simulink model "scattering_FP"  (R2021b)
settings: Solver=ode45  StartTime=0.0  StopTime=10  FixedStep=Ts  MinStep=1e-5  RelTol=1e-5
undefined symbols (not defined in the file): A, Ak, B, b, Be, Bh, Bs, C, d, Dh, Discrete, Dm, Ds, Fc, Fip, Flp, Jh, Ke, Kh, Ks, Mm, Ms, noise, Ph, R, Time, Ts, x0, xe
libraries: simulink x3, ctrlSharedLib x2, cstblocks x1
settings Model: Creator=simon  LastModifiedBy=buse
settings SolverCC: AlgebraicLoopSolver=LineSearch
settings DebuggingCC: SFMachineParentedDataDiag=warning

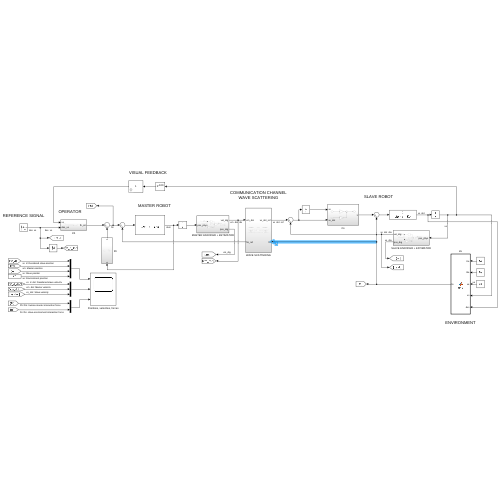
[thumbnail: Simulink's stored preview of the top-level diagram]
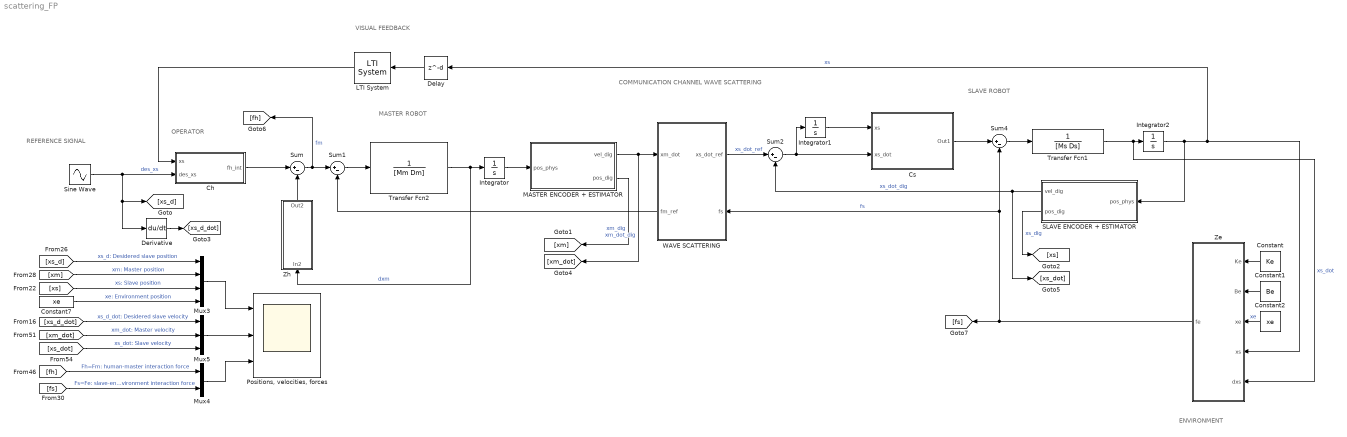
== system scattering_FP ==
  note: REFERENCE SIGNAL
  note: MASTER ROBOT
  note: COMMUNICATION CHANNEL
      | WAVE SCATTERING
  note: VISUAL FEEDBACK
  note: SLAVE ROBOT
  note: OPERATOR
  note: ENVIRONMENT
  Ch : Subsystem
  Constant : Constant  Value=Ke
  Constant1 : Constant  Value=Be
  Constant2 : Constant  Value=xe
  Constant7 : Constant  Value=xe
  Cs : Subsystem
  Delay : Delay  DelayLength=d
  Derivative : Derivative
  Integrator : Integrator
  Integrator1 : Integrator
  Integrator2 : Integrator
  LTI System : cstblocks/LTI System  sys=1  IC=[]
  MASTER ENCODER + ESTIMATOR : Subsystem
  Mux3 : Mux
  Mux4 : Mux  Inputs=2
  Mux5 : Mux  Inputs=3
  "Positions, velocities, forces" : Scope  NumInputPorts=3
  SLAVE ENCODER + ESTIMATOR : Subsystem
  Sine Wave : Sin  Amplitude=A  Frequency=Fc  SampleTime=0
  Sum{,1..2,4} (4 alike) : Sum  Inputs=|+-
  Transfer Fcn1 : TransferFcn  Denominator=[Ms Ds]
  Transfer Fcn2 : TransferFcn  Denominator=[Mm Dm]
  WAVE SCATTERING : Subsystem
      settings: PortSchema="{\"entries\":[{\"content\":{\"sides\":[{\"content\":{\"connectorIds\":[\"In1\",\"Out2\"]},\"type\":\"ConnectorPlacement.EquallySpacedRectSide\",\"uuid\":\"b52b5263-ec77-4a5b-a444-fedf8384a1f4\"},{\"content\":{\"connectorIds\":[\"Out1\",\"In2\"],\"side\":\"RIGHT\"},\"type\":\"ConnectorPlacement.EquallySpacedRectSide\",\"uuid\":\"29fc6d0d-53a2-4de5-b8fc-fdc6e2130f9a\"},{\"content\":{\"connectorIds\":[],\"side\":\"TOP\"},\"type\":\"ConnectorPlacement.EquallySpacedRectSide\",\"uuid\":\"d00abe1a-0b08-4fbd-831b-b235aed68611\"},{\"content\":{\"connectorIds\":[],\"side\":\"HIDDEN\"},\"type\":\"ConnectorPlacement.EquallySpacedRectSide\",\"uuid\":\"d0d3daa3-ebbf-4bb5-b3d9-7ef522d44ef5\"}]},\"type\":\"ConnectorPlacement.EquallySpacedConnector\",\"uuid\":\"e5a03f62-d534-4700-82c8-2ace6ee2abeb\"}],\"packageUris\":[\"http://schema.mathworks.com/mf0/Connector/R2020b\"],\"version\":\"1.0\"}"
  Ze : MATLAB Function  TreatAsAtomicUnit=on
  Zh : Subsystem
  wires:
  Zh/1(Out2) -> Sum/2
  Sum1/1 -> Transfer Fcn2/1
  Sum4/1 -> Transfer Fcn1/1
  Transfer Fcn1/1 -> Ze/5(dxs), Integrator2/1  "xs_dot"
  Integrator2/1 -> SLAVE ENCODER + ESTIMATOR/1(pos_phys), Ze/4(xs), Delay/1  "xs"
  Constant2/1 -> Ze/3(xe)  "xe"
  Constant1/1 -> Ze/2(Be)
  Constant/1 -> Ze/1(Ke)
  Sum/1 -> [fh], Sum1/1  "fm"
  WAVE SCATTERING/2(fm_ref) -> Sum1/2
  WAVE SCATTERING/1(xs_dot_ref) -> Sum2/1  "xs_dot_ref"
  Sum2/1 -> Integrator1/1, Cs/2(xs_dot)
  Integrator1/1 -> Cs/1(xs)
  Cs/1(Out1) -> Sum4/1
  MASTER ENCODER + ESTIMATOR/1(vel_dig) -> [xm_dot], WAVE SCATTERING/1(xm_dot)  "xm_dot_dig"
  Ch/1(fh_int) -> Sum/1
  LTI System/1 -> Ch/1(xs)
  SLAVE ENCODER + ESTIMATOR/1(vel_dig) -> [xs_dot], Sum2/2  "xs_dot_dig"
  Ze/1(fe) -> [fs], WAVE SCATTERING/2(fs), Sum4/2  "fs"
  Sine Wave/1 -> Derivative/1, [xs_d], Ch/2(des_xs)  "des_xs"
  Delay/1 -> LTI System/1
  [fs] -> Mux4/2  "Fs=Fe: slave-environment interaction force"
  [xm_dot] -> Mux5/2  "xm_dot: Master velocity"
  [xs_d] -> Mux3/1  "xs_d: Desidered slave position"
  [fh] -> Mux4/1  "Fh=Fm: human-master interaction force"
  [xs_dot] -> Mux5/3  "xs_dot: Slave velocity"
  [xs_d_dot] -> Mux5/1  "xs_d_dot: Desidered slave velocity"
  Mux5/1 -> "Positions, velocities, forces"/2
  Mux3/1 -> "Positions, velocities, forces"/1
  Mux4/1 -> "Positions, velocities, forces"/3
  [xm] -> Mux3/2  "xm: Master position"
  [xs] -> Mux3/3  "xs: Slave position"
  Constant7/1 -> Mux3/4  "xe: Environment position"
  MASTER ENCODER + ESTIMATOR/2(pos_dig) -> [xm]  "xm_dig"
  SLAVE ENCODER + ESTIMATOR/2(pos_dig) -> [xs]  "xs_dig"
  Derivative/1 -> [xs_d_dot]
  Transfer Fcn2/1 -> Integrator/1, Zh/1(In2)  "dxm"
  Integrator/1 -> MASTER ENCODER + ESTIMATOR/1(pos_phys)

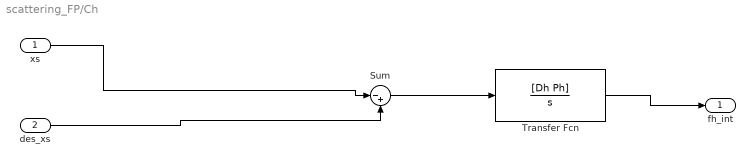
== system scattering_FP/Ch ==
  xs : Inport
  des_xs : Inport  Port=2
  Sum : Sum  Inputs=|-+
  Transfer Fcn : TransferFcn  Numerator=[Dh Ph]  Denominator=[1 0]
  fh_int : Outport
  wires:
  xs/1 -> Sum/1
  des_xs/1 -> Sum/2
  Sum/1 -> Transfer Fcn/1
  Transfer Fcn/1 -> fh_int/1

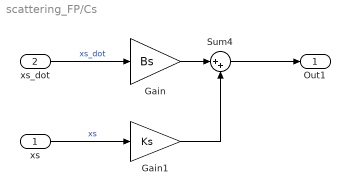
== system scattering_FP/Cs ==
  xs : Inport
  xs_dot : Inport  Port=2
  Gain : Gain  Gain=Bs
  Gain1 : Gain  Gain=Ks
  Sum4 : Sum  Inputs=|++
  Out1 : Outport
  wires:
  Gain1/1 -> Sum4/2
  Sum4/1 -> Out1/1
  xs_dot/1 -> Gain/1  "xs_dot"
  Gain/1 -> Sum4/1
  xs/1 -> Gain1/1  "xs"

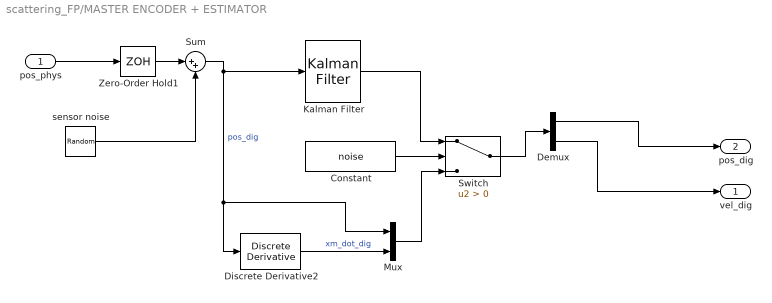
== system scattering_FP/MASTER ENCODER + ESTIMATOR ==
  pos_phys : Inport
  Constant : Constant  Value=noise
  Demux : Demux  Outputs=2
  Discrete Derivative2 : simulink/Discrete/Discrete Derivative  gainval=1.0  ICPrevScaledInput=0.0  OutMin=[]  OutMax=[]  OutDataType=fixdt(1, 16)  OutScaling=2^-10  DoSatur=off
  Kalman Filter : ctrlSharedLib/Kalman Filter  TimeDomain=Discrete-Time  UseCurrentEstimator=on  ModelSource=Individual A, B, C, D matrices  ModelSourceVariable=ss(0.95,1,1,0,1)  A=Ak  B=B  C=C  D=0  NumberOfStates=2  NumberOfInputs=1  NumberOfOutputs=1  InitialEstimateSource=Dialog  X0=x0  P0=10  UseK=off  UseGH=off  NumberOfProcessNoiseInputs=1  G=1  TimeInvariantG=on  H=0  TimeInvariantH=on  Q=Q_m  TimeInvariantQ=on  R=R  TimeInvariantR=on  N=0  TimeInvariantN=on  AddInputPort=off  AddEnablePort=off  OutputEstimatedY=off  OutputP=off  Ts=Ts
  Mux : Mux  Inputs=2
  Sum : Sum  Inputs=|++
  Switch : Switch  Criteria=u2 > Threshold
  Zero-Order Hold1 : ZeroOrderHold  SampleTime=Ts
  sensor noise : RandomNumber  Variance=noise  SampleTime=Ts
  vel_dig : Outport
  pos_dig : Outport  Port=2
  wires:
  pos_phys/1 -> Zero-Order Hold1/1
  Zero-Order Hold1/1 -> Sum/1
  sensor noise/1 -> Sum/2
  Kalman Filter/1 -> Switch/1
  Sum/1 -> Mux/1, Discrete Derivative2/1, Kalman Filter/1  "pos_dig"
  Constant/1 -> Switch/2
  Mux/1 -> Switch/3
  Discrete Derivative2/1 -> Mux/2  "xm_dot_dig"
  Switch/1 -> Demux/1
  Demux/1 -> pos_dig/1
  Demux/2 -> vel_dig/1

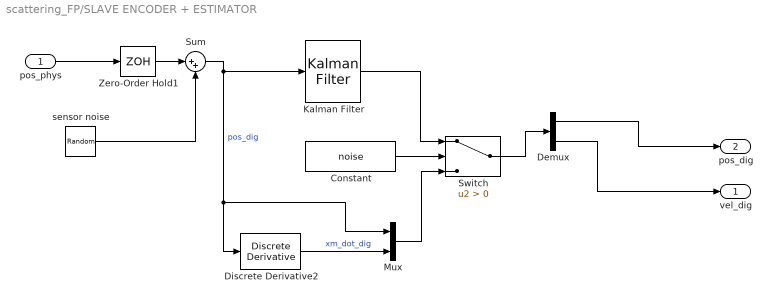
== system scattering_FP/SLAVE ENCODER + ESTIMATOR ==
  pos_phys : Inport
  Constant : Constant  Value=noise
  Demux : Demux  Outputs=2
  Discrete Derivative2 : simulink/Discrete/Discrete Derivative  gainval=1.0  ICPrevScaledInput=0.0  OutMin=[]  OutMax=[]  OutDataType=fixdt(1, 16)  OutScaling=2^-10  DoSatur=off
  Kalman Filter : ctrlSharedLib/Kalman Filter  TimeDomain=Discrete-Time  UseCurrentEstimator=on  ModelSource=Individual A, B, C, D matrices  ModelSourceVariable=ss(0.95,1,1,0,1)  A=Ak  B=B  C=C  D=0  NumberOfStates=2  NumberOfInputs=1  NumberOfOutputs=1  InitialEstimateSource=Dialog  X0=0  P0=10  UseK=off  UseGH=off  NumberOfProcessNoiseInputs=1  G=1  TimeInvariantG=on  H=0  TimeInvariantH=on  Q=Q_m  TimeInvariantQ=on  R=R  TimeInvariantR=on  N=0  TimeInvariantN=on  AddInputPort=off  AddEnablePort=off  OutputEstimatedY=off  OutputP=off  Ts=Ts
  Mux : Mux  Inputs=2
  Sum : Sum  Inputs=|++
  Switch : Switch  Criteria=u2 > Threshold
  Zero-Order Hold1 : ZeroOrderHold  SampleTime=Ts
  sensor noise : RandomNumber  Variance=noise  SampleTime=Ts
  vel_dig : Outport
  pos_dig : Outport  Port=2
  wires:
  pos_phys/1 -> Zero-Order Hold1/1
  Zero-Order Hold1/1 -> Sum/1
  sensor noise/1 -> Sum/2
  Kalman Filter/1 -> Switch/1
  Sum/1 -> Mux/1, Discrete Derivative2/1, Kalman Filter/1  "pos_dig"
  Constant/1 -> Switch/2
  Mux/1 -> Switch/3
  Discrete Derivative2/1 -> Mux/2  "xm_dot_dig"
  Switch/1 -> Demux/1
  Demux/1 -> pos_dig/1
  Demux/2 -> vel_dig/1

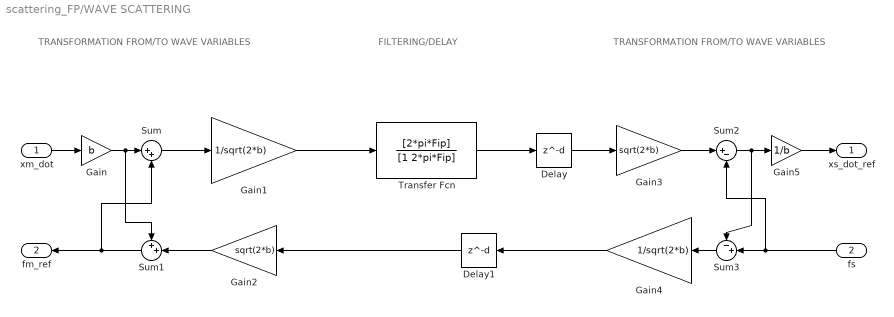
== system scattering_FP/WAVE SCATTERING ==
  note: FILTERING/DELAY
  note: TRANSFORMATION FROM/TO
      | WAVE VARIABLES
  note: TRANSFORMATION FROM/TO
      | WAVE VARIABLES
  xm_dot : Inport
  fs : Inport  Port=2
  Delay : Delay  DelayLength=d
  Delay1 : Delay  DelayLength=d
  Gain : Gain  Gain=b
  Gain1 : Gain  Gain=1/sqrt(2*b)
  Gain2 : Gain  Gain=sqrt(2*b)
  Gain3 : Gain  Gain=sqrt(2*b)
  Gain4 : Gain  Gain=1/sqrt(2*b)
  Gain5 : Gain  Gain=1/b
  Sum : Sum  Inputs=|++
  Sum1 : Sum  Inputs=++|
  Sum2 : Sum  Inputs=|+-
  Sum3 : Sum  Inputs=-+|
  Transfer Fcn : TransferFcn  Numerator=[2*pi*Fip]  Denominator=[1 2*pi*Fip]
  xs_dot_ref : Outport
  fm_ref : Outport  Port=2
  wires:
  xm_dot/1 -> Gain/1
  Gain/1 -> Sum1/1, Sum/1
  Sum/1 -> Gain1/1
  Sum1/1 -> Sum/2, fm_ref/1
  Gain2/1 -> Sum1/2
  Gain1/1 -> Transfer Fcn/1
  Transfer Fcn/1 -> Delay/1
  Delay1/1 -> Gain2/1
  Delay/1 -> Gain3/1
  Gain3/1 -> Sum2/1
  Sum3/1 -> Gain4/1
  Gain4/1 -> Delay1/1
  Sum2/1 -> Sum3/1, Gain5/1
  Gain5/1 -> xs_dot_ref/1
  fs/1 -> Sum3/2, Sum2/2

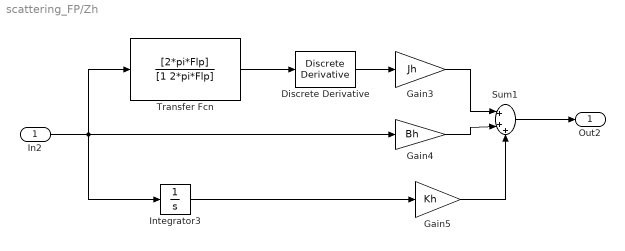
== system scattering_FP/Zh ==
  In2 : Inport
  Discrete Derivative : simulink/Discrete/Discrete Derivative  gainval=1.0  ICPrevScaledInput=0.0  OutMin=[]  OutMax=[]  OutDataType=fixdt(1, 16)  OutScaling=2^-10  DoSatur=off
  Gain3 : Gain  Gain=Jh
  Gain4 : Gain  Gain=Bh
  Gain5 : Gain  Gain=Kh
  Integrator3 : Integrator
  Sum1 : Sum  Inputs=|+++
  Transfer Fcn : TransferFcn  Numerator=[2*pi*Flp]  Denominator=[1 2*pi*Flp]
  Out2 : Outport
  wires:
  Sum1/1 -> Out2/1
  Gain4/1 -> Sum1/2
  Gain5/1 -> Sum1/3
  In2/1 -> Transfer Fcn/1, Integrator3/1, Gain4/1
  Gain3/1 -> Sum1/1
  Integrator3/1 -> Gain5/1
  Discrete Derivative/1 -> Gain3/1
  Transfer Fcn/1 -> Discrete Derivative/1

== matlab function scattering_FP/Ze ==
  data: Ke input; fe output; Be input; xe input; xs input; dxs input
function fe = env(Ke, Be, xe, xs, dxs)
    if xs > xe
        fe = Ke*(xs-xe)+Be*max(dxs, 0);
    else
        fe = 0;
    end
